simulink model "F16_actlib"  (R2018b)
settings: Solver=ode45  StartTime=0.0  StopTime=10.0  RelTol=1e-3  EnableMultiTasking=on
values from neighbouring files (symbols this model uses):
  init_dlef = dLEF    [FindF16Dynamics.m]    (also in runF16model.m = uu(5))
  init_u = [trim_thrust_lo;trim_control_lo]    [FindF16Dynamics.m]    (also in runF16model.m = uu(1:4))
settings Model: Creator=LXS  LastModifiedBy=LXS
settings DataIOCC: LimitDataPoints=on  SaveFormat=Array  SignalLoggingSaveFormat=ModelDataLogs
settings OptimizationCC: InitFltsAndDblsToZero=on  LifeSpan=inf
settings DebuggingCC: SaveWithParameterizedLinksMsg=none  UnderspecifiedInitializationDetection=Classic  MergeDetectMultiDrivingBlocksExec=none  SignalResolutionControl=TryResolveAllWithWarning  SolverPrmCheckMsg=warning  MultiTaskDSMMsg=warning  MultiTaskCondExecSysMsg=none  SFUnexpectedBacktrackingDiag=warning  SFNoUnconditionalDefaultTransitionDiag=warning  SFExecutionAtInitializationDiag=none
settings HardwareCC: ProdBitPerPointer=32  ProdBitPerSizeT=32  ProdBitPerPtrDiffT=32  ProdLargestAtomicFloat=None  ProdIntDivRoundTo=Undefined  ProdEndianess=Unspecified  ProdWordSize=32  ProdHWDeviceType=32-bit Generic
settings ModelReferenceCC: PropagateSignalLabelsOutOfModel=off
settings SFSimCC: SimParseCustomCode=off
settings CodeAppCC: StateflowObjectComments=on
settings GRTTargetCC: TargetFcnLib=ansi_tfl_tmw.mat  TargetLangStandard=C89/C90 (ANSI)  CombineOutputUpdateFcns=off  GRTInterface=on
settings ConfigComp: CovMetricSettings=dw  CovHtmlReporting=on  CovSaveCumulativeToWorkspaceVar=on  CovSaveSingleToWorkspaceVar=on

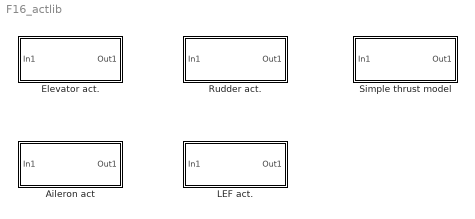
== system F16_actlib ==
  Aileron act : Subsystem
      mask Display:
      | port_label('output', 1, 'da')
      | port_label('input', 1, 'da_ref')
  Elevator act. : Subsystem
      mask Display:
      | port_label('output', 1, 'de')
      | port_label('input', 1, 'de_ref')
  LEF act. : Subsystem
      mask Display:
      | port_label('output', 1, 'dlef')
      | port_label('input', 1, 'dlef_ref')
  Rudder act. : Subsystem
      mask Display:
      | port_label('output', 1, 'dr')
      | port_label('input', 1, 'dr_ref')
  Simple thrust model : Subsystem
      mask Display:
      | port_label('output', 1, 'T')
      | port_label('input', 1, 'T_ref')

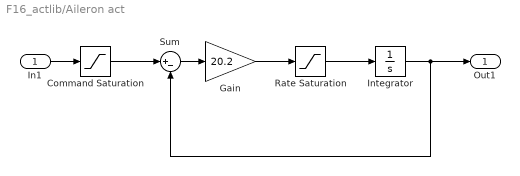
== system F16_actlib/Aileron act ==
  In1 : Inport
  Command Saturation : Saturate  UpperLimit=21.5*pi/180  LowerLimit=-21.5*pi/180
  Gain : Gain  Gain=20.2  SaturateOnIntegerOverflow=on  OutDataTypeStr=Inherit: Same as input  ParamDataTypeStr=Inherit: Same as input
  "Integrator " : Integrator  InitialCondition=init_u(3)  UpperSaturationLimit=21.5  LowerSaturationLimit=-21.5
  Rate Saturation : Saturate  UpperLimit=80*pi/180  LowerLimit=-80*pi/180
  Sum : Sum  Inputs=|+-  SaturateOnIntegerOverflow=on  InputSameDT=on  OutDataTypeStr=Inherit: Same as first input
  Out1 : Outport
  wires:
  In1/1 -> Command Saturation/1
  Command Saturation/1 -> Sum/1
  Sum/1 -> Gain/1
  Gain/1 -> Rate Saturation/1
  Rate Saturation/1 -> "Integrator "/1
  "Integrator "/1 -> Out1/1, Sum/2

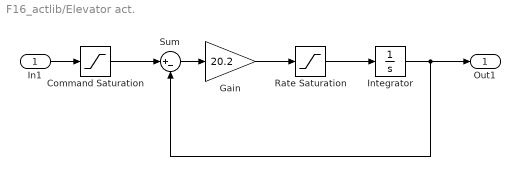
== system F16_actlib/Elevator act. ==
  In1 : Inport
  Command Saturation : Saturate  UpperLimit=25*pi/180  LowerLimit=-25*pi/180
  Gain : Gain  Gain=20.2  SaturateOnIntegerOverflow=on  OutDataTypeStr=Inherit: Same as input  ParamDataTypeStr=Inherit: Same as input
  "Integrator " : Integrator  InitialCondition=init_u(2)  UpperSaturationLimit=25  LowerSaturationLimit=-25
  Rate Saturation : Saturate  UpperLimit=60*pi/180  LowerLimit=-60*pi/180
  Sum : Sum  Inputs=|+-  SaturateOnIntegerOverflow=on  InputSameDT=on  OutDataTypeStr=Inherit: Same as first input
  Out1 : Outport
  wires:
  In1/1 -> Command Saturation/1
  Command Saturation/1 -> Sum/1
  Sum/1 -> Gain/1
  Gain/1 -> Rate Saturation/1
  Rate Saturation/1 -> "Integrator "/1
  "Integrator "/1 -> Out1/1, Sum/2

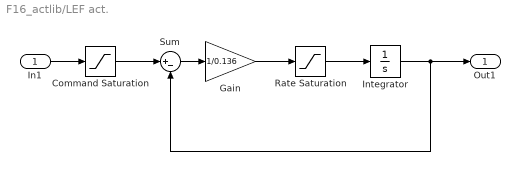
== system F16_actlib/LEF act. ==
  In1 : Inport
  Command Saturation : Saturate  UpperLimit=25  LowerLimit=0
  Gain : Gain  Gain=1/0.136  SaturateOnIntegerOverflow=on  OutDataTypeStr=Inherit: Same as input  ParamDataTypeStr=Inherit: Same as input
  "Integrator " : Integrator  InitialCondition=init_dlef  UpperSaturationLimit=25  LowerSaturationLimit=-25
  Rate Saturation : Saturate  UpperLimit=25  LowerLimit=-25
  Sum : Sum  Inputs=|+-  SaturateOnIntegerOverflow=on  InputSameDT=on  OutDataTypeStr=Inherit: Same as first input
  Out1 : Outport
  wires:
  "Integrator "/1 -> Sum/2, Out1/1
  Rate Saturation/1 -> "Integrator "/1
  Gain/1 -> Rate Saturation/1
  Sum/1 -> Gain/1
  Command Saturation/1 -> Sum/1
  In1/1 -> Command Saturation/1

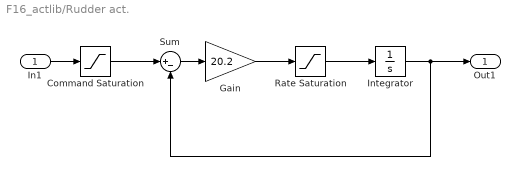
== system F16_actlib/Rudder act. ==
  In1 : Inport
  Command Saturation : Saturate  UpperLimit=30*pi/180  LowerLimit=-30*pi/180
  Gain : Gain  Gain=20.2  SaturateOnIntegerOverflow=on  OutDataTypeStr=Inherit: Same as input  ParamDataTypeStr=Inherit: Same as input
  "Integrator " : Integrator  InitialCondition=init_u(4)  UpperSaturationLimit=25  LowerSaturationLimit=-25
  Rate Saturation : Saturate  UpperLimit=120*pi/180  LowerLimit=-120*pi/180
  Sum : Sum  Inputs=|+-  SaturateOnIntegerOverflow=on  InputSameDT=on  OutDataTypeStr=Inherit: Same as first input
  Out1 : Outport
  wires:
  "Integrator "/1 -> Sum/2, Out1/1
  Rate Saturation/1 -> "Integrator "/1
  Gain/1 -> Rate Saturation/1
  Sum/1 -> Gain/1
  Command Saturation/1 -> Sum/1
  In1/1 -> Command Saturation/1

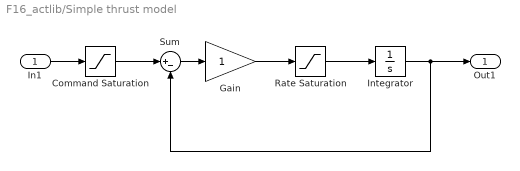
== system F16_actlib/Simple thrust model ==
  In1 : Inport
  Command Saturation : Saturate  UpperLimit=85000  LowerLimit=4500
  Gain : Gain  SaturateOnIntegerOverflow=on  OutDataTypeStr=Inherit: Same as input  ParamDataTypeStr=Inherit: Same as input
  "Integrator " : Integrator  InitialCondition=init_u(1)  UpperSaturationLimit=45000  LowerSaturationLimit=-45000
  Rate Saturation : Saturate  UpperLimit=45000  LowerLimit=-45000
  Sum : Sum  Inputs=|+-  SaturateOnIntegerOverflow=on  InputSameDT=on  OutDataTypeStr=Inherit: Same as first input
  Out1 : Outport
  wires:
  In1/1 -> Command Saturation/1
  Command Saturation/1 -> Sum/1
  Sum/1 -> Gain/1
  Gain/1 -> Rate Saturation/1
  Rate Saturation/1 -> "Integrator "/1
  "Integrator "/1 -> Out1/1, Sum/2
